simulink model "GalvoModel_servolike_v2_simpli_B"  (R2013a)
settings: Solver=ode45  StartTime=0.0  StopTime=10.0  RelTol=1e-3
values from neighbouring files (symbols this model uses):
  BEM = 108e-6    (= 0.000108)    [GalvoModel_WOK_step.m]
  KTR = 47e-3    (= 0.047)    [GalvoModel_WOK_step.m]
  T1 = R1*C1    (= 0.000264)    [GalvoModel_v6_sys.m]
undefined symbols (not defined in the file or in its folder): K1, K2, T2
settings Model: Creator=mainster  LastModifiedBy=mainster
settings DebuggingCC: SolverPrmCheckMsg=none  InitInArrayFormatMsg=none

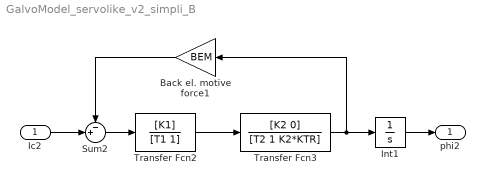
== system GalvoModel_servolike_v2_simpli_B ==
  Ic2 : Inport
  Back el. motive force1 : Gain  Gain=BEM
  Int1 : Integrator
  Sum2 : Sum  Inputs=-+|
  Transfer Fcn2 : TransferFcn  Numerator=[K1]  Denominator=[T1 1]
  Transfer Fcn3 : TransferFcn  Numerator=[K2 0]  Denominator=[T2 1 K2*KTR]
  phi2 : Outport
  wires:
  Ic2/1 -> Sum2/2
  Sum2/1 -> Transfer Fcn2/1
  Transfer Fcn3/1 -> Int1/1, Back el. motive force1/1
  Int1/1 -> phi2/1
  Back el. motive force1/1 -> Sum2/1
  Transfer Fcn2/1 -> Transfer Fcn3/1
